simulink model "IIRFilterMapping_dsp2"  (R2016b)
settings: Solver=FixedStepAuto  StartTime=0.0  StopTime=100  FixedStep=1  RelTol=1e-3
undefined symbols (not defined in the file or in its folder): a, b
settings Model: Creator=Jelena  LastModifiedBy=Jelena

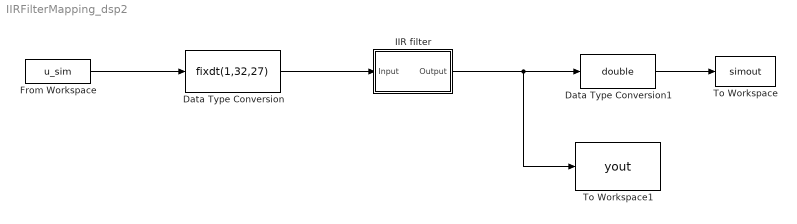
== system IIRFilterMapping_dsp2 ==
  Data Type Conversion : DataTypeConversion  OutDataTypeStr=fixdt(1,32,27)  RndMeth=Round
  Data Type Conversion1 : DataTypeConversion  OutDataTypeStr=double  RndMeth=Round
  From Workspace : FromWorkspace  VariableName=u_sim
  IIR filter : Subsystem  Tag=FilterWizardSubSystem
  To Workspace : ToWorkspace  VariableName=simout  SaveFormat=Timeseries  SampleTime=-1
  To Workspace1 : ToWorkspace  VariableName=yout  SampleTime=-1
  wires:
  IIR filter/1(Output) -> To Workspace1/1, Data Type Conversion1/1
  Data Type Conversion1/1 -> To Workspace/1
  Data Type Conversion/1 -> IIR filter/1(Input)
  From Workspace/1 -> Data Type Conversion/1

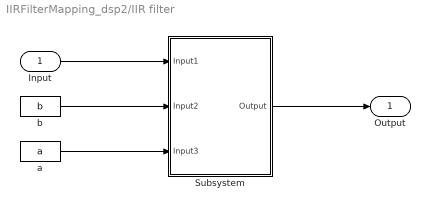
== system IIRFilterMapping_dsp2/IIR filter ==
  Input : Inport
  Subsystem : Subsystem  Tag=FilterWizardSubSystem
      settings: ErrorFcn=dspFilterRealizedInBasicElemsAlgLoopErrFcnCallback
  a : Constant  Value=a  VectorParams1D=off  OutDataTypeStr=fixdt(1,32,27)
  b : Constant  Value=b  VectorParams1D=off  OutDataTypeStr=fixdt(1,32,27)
  Output : Outport  OutDataTypeStr=fixdt(1,32,27)
  wires:
  Input/1 -> Subsystem/1(Input1)
  b/1 -> Subsystem/2(Input2)
  a/1 -> Subsystem/3(Input3)
  Subsystem/1(Output) -> Output/1

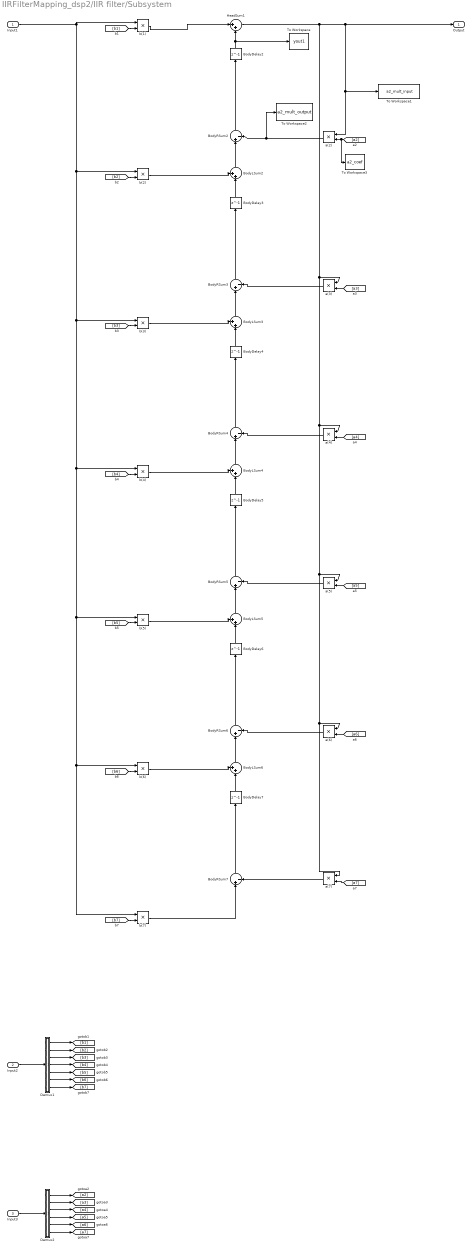
== system IIRFilterMapping_dsp2/IIR filter/Subsystem ==
  Input1 : Inport
  Input2 : Inport  Port=2
  Input3 : Inport  Port=3
  BodyDelay{2..7} (6 alike) : Delay  DelayLength=1  InitialCondition=0
  BodyLSum{2..6} (5 alike) : Sum  Inputs=++|  RndMeth=Nearest  SaturateOnIntegerOverflow=on  OutDataTypeStr=Inherit: Same as first input
  BodyRSum2 : Sum  Inputs=|+-  AccumDataTypeStr=fixdt(1,32,27)  OutDataTypeStr=fixdt(1,32,27)  RndMeth=Round  SaturateOnIntegerOverflow=on
  BodyRSum{3..7} (5 alike) : Sum  Inputs=|+-  RndMeth=Nearest  SaturateOnIntegerOverflow=on  OutDataTypeStr=Inherit: Same as first input
  Demux1 : Subsystem
  Demux2 : Subsystem
  HeadSum1 : Sum  Inputs=|++  AccumDataTypeStr=fixdt(1,32,27)  OutDataTypeStr=fixdt(1,32,27)  RndMeth=Nearest  SaturateOnIntegerOverflow=on
  To Workspace : ToWorkspace  VariableName=yout1  SampleTime=-1
  To Workspace1 : ToWorkspace  VariableName=a2_mult_input  SampleTime=-1
      settings: Save2DSignal=2-D array (concatenate along first dimension)
  To Workspace2 : ToWorkspace  VariableName=a2_mult_output  SampleTime=-1
      settings: Save2DSignal=2-D array (concatenate along first dimension)
  To Workspace3 : ToWorkspace  VariableName=a2_coef  SampleTime=-1
      settings: Save2DSignal=2-D array (concatenate along first dimension)
  a(2) : Product  OutDataTypeStr=fixdt(1,32,27)  RndMeth=Round  SaturateOnIntegerOverflow=on
  a(3) : Product  RndMeth=Nearest  SaturateOnIntegerOverflow=on  OutDataTypeStr=Inherit: Same as first input
  a(4) : Product  RndMeth=Nearest  SaturateOnIntegerOverflow=on  OutDataTypeStr=Inherit: Same as first input
  a(5) : Product  RndMeth=Nearest  SaturateOnIntegerOverflow=on  OutDataTypeStr=Inherit: Same as first input
  a(6) : Product  RndMeth=Nearest  SaturateOnIntegerOverflow=on  OutDataTypeStr=Inherit: Same as first input
  a(7) : Product  RndMeth=Nearest  SaturateOnIntegerOverflow=on  OutDataTypeStr=Inherit: Same as first input
  b(1) : Product  RndMeth=Nearest  SaturateOnIntegerOverflow=on  OutDataTypeStr=Inherit: Same as first input
  b(2) : Product  RndMeth=Nearest  SaturateOnIntegerOverflow=on  OutDataTypeStr=Inherit: Same as first input
  b(3) : Product  RndMeth=Nearest  SaturateOnIntegerOverflow=on  OutDataTypeStr=Inherit: Same as first input
  b(4) : Product  RndMeth=Nearest  SaturateOnIntegerOverflow=on  OutDataTypeStr=Inherit: Same as first input
  b(5) : Product  RndMeth=Nearest  SaturateOnIntegerOverflow=on  OutDataTypeStr=Inherit: Same as first input
  b(6) : Product  RndMeth=Nearest  SaturateOnIntegerOverflow=on  OutDataTypeStr=Inherit: Same as first input
  b(7) : Product  RndMeth=Nearest  SaturateOnIntegerOverflow=on  OutDataTypeStr=Inherit: Same as first input
  Output : Outport
  wires:
  [b1] -> b(1)/2
  [b2] -> b(2)/2
  [a2] -> To Workspace3/1, a(2)/2
  [b3] -> b(3)/2
  [a3] -> a(3)/2
  [b4] -> b(4)/2
  [a4] -> a(4)/2
  [b5] -> b(5)/2
  [a5] -> a(5)/2
  [b6] -> b(6)/2
  [a6] -> a(6)/2
  [b7] -> b(7)/2
  [a7] -> a(7)/2
  Demux1/1(output1) -> [b1]
  Demux1/2(output2) -> [b2]
  Demux1/3(output3) -> [b3]
  Demux1/4(output4) -> [b4]
  Demux1/5(output5) -> [b5]
  Demux1/6(output6) -> [b6]
  Demux1/7(output7) -> [b7]
  Demux2/1(output1) -> [a2]
  Demux2/2(output2) -> [a3]
  Demux2/3(output3) -> [a4]
  Demux2/4(output4) -> [a5]
  Demux2/5(output5) -> [a6]
  Demux2/6(output6) -> [a7]
  Input1/1 -> b(6)/1, b(7)/1, b(5)/1, b(4)/1, b(3)/1, b(2)/1, b(1)/1
  b(1)/1 -> HeadSum1/1
  b(2)/1 -> BodyLSum2/1
  BodyLSum2/1 -> BodyRSum2/1
  BodyRSum2/1 -> BodyDelay2/1
  a(2)/1 -> To Workspace2/1, BodyRSum2/2
  BodyDelay2/1 -> To Workspace/1, HeadSum1/2
  b(3)/1 -> BodyLSum3/1
  BodyLSum3/1 -> BodyRSum3/1
  BodyRSum3/1 -> BodyDelay3/1
  a(3)/1 -> BodyRSum3/2
  BodyDelay3/1 -> BodyLSum2/2
  b(4)/1 -> BodyLSum4/1
  BodyLSum4/1 -> BodyRSum4/1
  BodyRSum4/1 -> BodyDelay4/1
  a(4)/1 -> BodyRSum4/2
  BodyDelay4/1 -> BodyLSum3/2
  b(5)/1 -> BodyLSum5/1
  BodyLSum5/1 -> BodyRSum5/1
  BodyRSum5/1 -> BodyDelay5/1
  a(5)/1 -> BodyRSum5/2
  BodyDelay5/1 -> BodyLSum4/2
  b(6)/1 -> BodyLSum6/1
  BodyLSum6/1 -> BodyRSum6/1
  BodyRSum6/1 -> BodyDelay6/1
  a(6)/1 -> BodyRSum6/2
  BodyDelay6/1 -> BodyLSum5/2
  b(7)/1 -> BodyRSum7/1
  BodyRSum7/1 -> BodyDelay7/1
  a(7)/1 -> BodyRSum7/2
  BodyDelay7/1 -> BodyLSum6/2
  Input2/1 -> Demux1/1(input)
  Input3/1 -> Demux2/1(input)
  HeadSum1/1 -> a(6)/1, a(7)/1, a(5)/1, a(4)/1, a(3)/1, Output/1, To Workspace1/1, a(2)/1

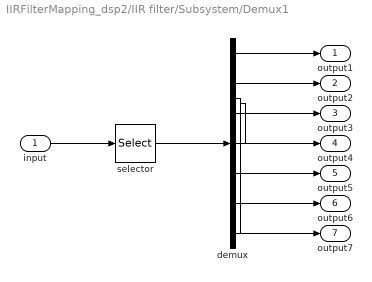
== system IIRFilterMapping_dsp2/IIR filter/Subsystem/Demux1 ==
  input : Inport
  demux : Demux  Outputs=7
  selector : Selector  InputPortWidth=7  IndexOptions=Index vector (dialog)  Indices=[1 2 3 4 5 6 7]  OutputSizes=1
  output1 : Outport
  output2 : Outport  Port=2
  output3 : Outport  Port=3
  output4 : Outport  Port=4
  output5 : Outport  Port=5
  output6 : Outport  Port=6
  output7 : Outport  Port=7
  wires:
  demux/1 -> output1/1
  demux/2 -> output2/1
  demux/3 -> output3/1
  demux/4 -> output4/1
  demux/5 -> output5/1
  demux/6 -> output6/1
  demux/7 -> output7/1
  input/1 -> selector/1
  selector/1 -> demux/1

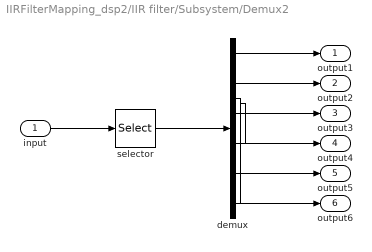
== system IIRFilterMapping_dsp2/IIR filter/Subsystem/Demux2 ==
  input : Inport
  demux : Demux  Outputs=6
  selector : Selector  InputPortWidth=7  IndexOptions=Index vector (dialog)  Indices=[2 3 4 5 6 7]  OutputSizes=1
  output1 : Outport
  output2 : Outport  Port=2
  output3 : Outport  Port=3
  output4 : Outport  Port=4
  output5 : Outport  Port=5
  output6 : Outport  Port=6
  wires:
  demux/1 -> output1/1
  demux/2 -> output2/1
  demux/3 -> output3/1
  demux/4 -> output4/1
  demux/5 -> output5/1
  demux/6 -> output6/1
  input/1 -> selector/1
  selector/1 -> demux/1
